simulink model "trefasstrommar"  (R2020a)
settings: Solver=FixedStepAuto  StartTime=0.0  StopTime=0.03  FixedStep=0.0001  RelTol=1e-3
values from neighbouring files (symbols this model uses):
  R = 40    [Forberedelser.m]    (also in Lab1.m = 881.666666667)
settings Model: Creator=Olof  LastModifiedBy=98all
settings SFSimCC: CustomCodeUndefinedFunction=UseInterfaceOnly

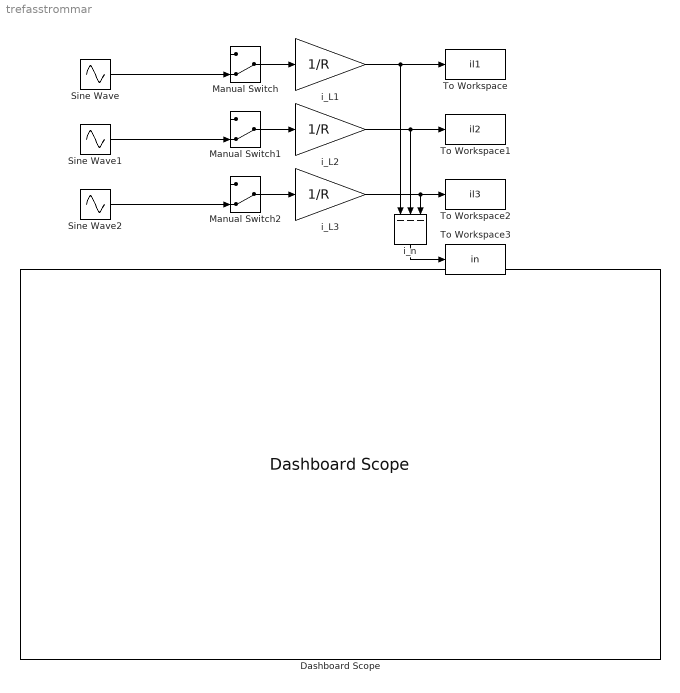
== system trefasstrommar ==
  Dashboard Scope : DashboardScope
  Manual Switch : ManualSwitch  CurrentSetting=0
  Manual Switch1 : ManualSwitch  CurrentSetting=0
  Manual Switch2 : ManualSwitch  CurrentSetting=0
  Sine Wave : Sin  Amplitude=sqrt(2)*127  Frequency=100*pi  SampleTime=0
  Sine Wave1 : Sin  Amplitude=sqrt(2)*127  Frequency=100*pi  Phase=-(2/3)*pi  SampleTime=0
  Sine Wave2 : Sin  Amplitude=sqrt(2)*127  Frequency=100*pi  Phase=-4*pi/3  SampleTime=0
  To Workspace : ToWorkspace  VariableName=il1  SaveFormat=Timeseries  SampleTime=-1
  To Workspace1 : ToWorkspace  VariableName=il2  SaveFormat=Timeseries  SampleTime=-1
  To Workspace2 : ToWorkspace  VariableName=il3  SaveFormat=Timeseries  SampleTime=-1
  To Workspace3 : ToWorkspace  VariableName=in  SaveFormat=Timeseries  SampleTime=-1
  i_L1 : Gain  Gain=1/R
  "i_L2 " : Gain  Gain=1/R
  i_L3 : Gain  Gain=1/R
  i_n : Sum  Inputs=---
  wires:
  Sine Wave/1 -> Manual Switch/2
  Sine Wave1/1 -> Manual Switch1/2
  Sine Wave2/1 -> Manual Switch2/2
  Manual Switch/1 -> i_L1/1
  Manual Switch1/1 -> "i_L2 "/1
  Manual Switch2/1 -> i_L3/1
  i_L1/1 -> i_n/1, To Workspace/1
  "i_L2 "/1 -> i_n/2, To Workspace1/1
  i_L3/1 -> i_n/3, To Workspace2/1
  i_n/1 -> To Workspace3/1
